simulink model "our_ch47"  (R2021a)
settings: Solver=FixedStepAuto  StartTime=0.0  StopTime=10  FixedStep=0.001  RelTol=1e-3  AbsTol=1e-3  EnableMultiTasking=on
undefined symbols (not defined in the file or in its folder): DiscIntNeverNeededParam, e2b, envs, PID_Param1, pos1, pos2, pos3, pos4, pos_load, tandem, X, x0, Y, Z
libraries: sm_lib x88, nesl_utility x25
(part 4 of 6)

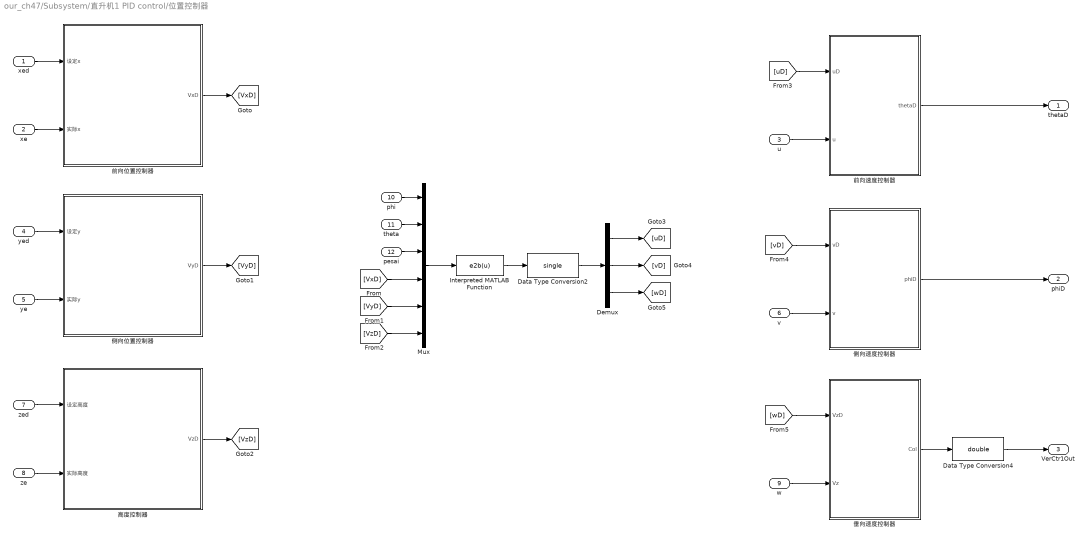
== system our_ch47/Subsystem/直升机1 PID control/位置控制器 ==
  xed : Inport
  xe : Inport  Port=2
  u : Inport  Port=3
  yed : Inport  Port=4
  ye : Inport  Port=5
  v : Inport  Port=6
  zed : Inport  Port=7
  ze : Inport  Port=8
  w : Inport  Port=9
  phi : Inport  Port=10
  theta : Inport  Port=11
  pesai : Inport  Port=12
  Data Type Conversion2 : DataTypeConversion  OutDataTypeStr=single  LockScale=on
  Data Type Conversion4 : DataTypeConversion  OutDataTypeStr=double  LockScale=on
  Demux : Demux  Outputs=3
  Interpreted MATLAB Function : MATLABFcn  MATLABFcn=e2b(u)  OutputDimensions=3
  Mux : Mux  Inputs=6
  侧向位置控制器 : Subsystem
  侧向速度控制器 : Subsystem
  前向位置控制器 : Subsystem
  前向速度控制器 : Subsystem
  垂向速度控制器 : Subsystem
  高度控制器 : Subsystem
  thetaD : Outport
  phiD : Outport  Port=2
  VerCtr1Out : Outport  Port=3
  wires:
  xe/1 -> 前向位置控制器/2(实际x)
  xed/1 -> 前向位置控制器/1(设定x)
  u/1 -> 前向速度控制器/2(u)
  前向速度控制器/1(thetaD) -> thetaD/1
  ye/1 -> 侧向位置控制器/2(实际y)
  yed/1 -> 侧向位置控制器/1(设定y)
  侧向速度控制器/1(phiD) -> phiD/1
  v/1 -> 侧向速度控制器/2(v)
  [wD] -> 垂向速度控制器/1(VzD)
  垂向速度控制器/1(Col) -> Data Type Conversion4/1
  w/1 -> 垂向速度控制器/2(Vz)
  Data Type Conversion4/1 -> VerCtr1Out/1
  zed/1 -> 高度控制器/1(设定高度)
  ze/1 -> 高度控制器/2(实际高度)
  前向位置控制器/1(VxD) -> [VxD]
  侧向位置控制器/1(VyD) -> [VyD]
  高度控制器/1(VzD) -> [VzD]
  theta/1 -> Mux/2
  phi/1 -> Mux/1
  pesai/1 -> Mux/3
  [VxD] -> Mux/4
  [VyD] -> Mux/5
  [VzD] -> Mux/6
  Interpreted MATLAB Function/1 -> Data Type Conversion2/1
  Demux/3 -> [wD]
  Demux/2 -> [vD]
  Demux/1 -> [uD]
  Data Type Conversion2/1 -> Demux/1
  Mux/1 -> Interpreted MATLAB Function/1
  [vD] -> 侧向速度控制器/1(vD)
  [uD] -> 前向速度控制器/1(uD)

== system our_ch47/Subsystem/直升机1 PID control/姿态控制器 ==
  RollD : Inport
  Roll : Inport  Port=2
  RollRate : Inport  Port=3
  PitchD : Inport  Port=4
  Pitch : Inport  Port=5
  PitchRate : Inport  Port=6
  YawD : Inport  Port=7
  Yaw : Inport  Port=8
  YawRate : Inport  Port=9
  Data Type Conversion1 : DataTypeConversion  OutDataTypeStr=double  LockScale=on
  Data Type Conversion2 : DataTypeConversion  OutDataTypeStr=double  LockScale=on
  Data Type Conversion3 : DataTypeConversion  OutDataTypeStr=double  LockScale=on
  俯仰控制器H-A : Subsystem
  滚转控制器H-A : Subsystem
  航向控制器H-A : Subsystem
  RollCtrlOut : Outport  VectorParamsAs1DForOutWhenUnconnected=off
  PitchCtrlOut : Outport  Port=2  VectorParamsAs1DForOutWhenUnconnected=off
  YawCtrlOut : Outport  Port=3  VectorParamsAs1DForOutWhenUnconnected=off
  wires:
  PitchRate/1 -> 俯仰控制器H-A/3(PitchRate)
  PitchD/1 -> 俯仰控制器H-A/1(PitchD)
  Pitch/1 -> 俯仰控制器H-A/2(Pitch)
  RollD/1 -> 滚转控制器H-A/1(RollD)
  Roll/1 -> 滚转控制器H-A/2(Roll)
  RollRate/1 -> 滚转控制器H-A/3(RollRate)
  YawRate/1 -> 航向控制器H-A/3(YawRate)
  YawD/1 -> 航向控制器H-A/1(YawD)
  Yaw/1 -> 航向控制器H-A/2(Yaw)
  俯仰控制器H-A/1(Lon) -> Data Type Conversion1/1
  航向控制器H-A/1(Ped) -> Data Type Conversion3/1
  滚转控制器H-A/1(Lat) -> Data Type Conversion2/1
  Data Type Conversion2/1 -> RollCtrlOut/1
  Data Type Conversion1/1 -> PitchCtrlOut/1
  Data Type Conversion3/1 -> YawCtrlOut/1

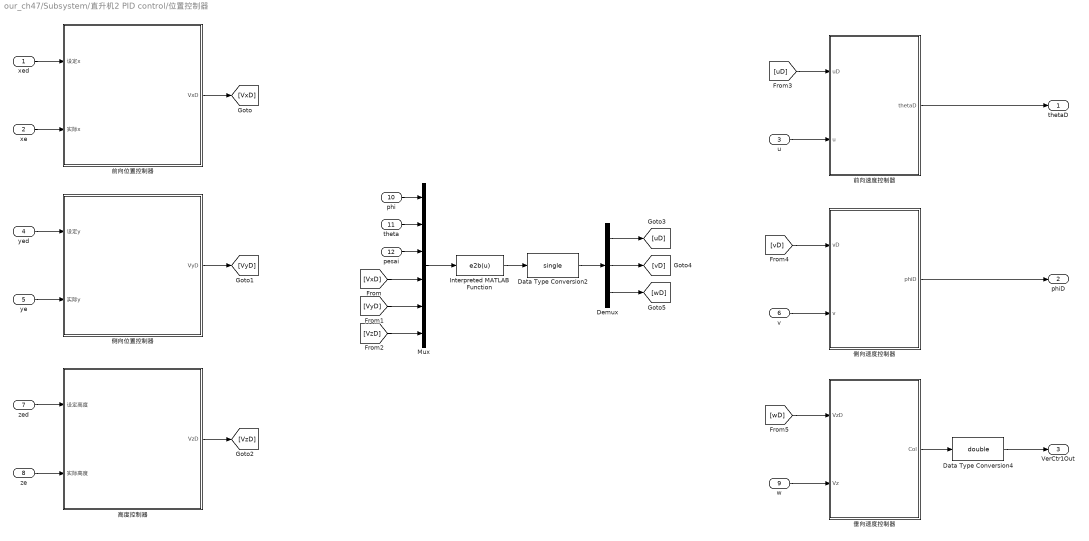
== system our_ch47/Subsystem/直升机2 PID control/位置控制器 ==
  xed : Inport
  xe : Inport  Port=2
  u : Inport  Port=3
  yed : Inport  Port=4
  ye : Inport  Port=5
  v : Inport  Port=6
  zed : Inport  Port=7
  ze : Inport  Port=8
  w : Inport  Port=9
  phi : Inport  Port=10
  theta : Inport  Port=11
  pesai : Inport  Port=12
  Data Type Conversion2 : DataTypeConversion  OutDataTypeStr=single  LockScale=on
  Data Type Conversion4 : DataTypeConversion  OutDataTypeStr=double  LockScale=on
  Demux : Demux  Outputs=3
  Interpreted MATLAB Function : MATLABFcn  MATLABFcn=e2b(u)  OutputDimensions=3
  Mux : Mux  Inputs=6
  侧向位置控制器 : Subsystem
  侧向速度控制器 : Subsystem
  前向位置控制器 : Subsystem
  前向速度控制器 : Subsystem
  垂向速度控制器 : Subsystem
  高度控制器 : Subsystem
  thetaD : Outport
  phiD : Outport  Port=2
  VerCtr1Out : Outport  Port=3
  wires:
  xe/1 -> 前向位置控制器/2(实际x)
  xed/1 -> 前向位置控制器/1(设定x)
  u/1 -> 前向速度控制器/2(u)
  前向速度控制器/1(thetaD) -> thetaD/1
  ye/1 -> 侧向位置控制器/2(实际y)
  yed/1 -> 侧向位置控制器/1(设定y)
  侧向速度控制器/1(phiD) -> phiD/1
  v/1 -> 侧向速度控制器/2(v)
  [wD] -> 垂向速度控制器/1(VzD)
  垂向速度控制器/1(Col) -> Data Type Conversion4/1
  w/1 -> 垂向速度控制器/2(Vz)
  Data Type Conversion4/1 -> VerCtr1Out/1
  zed/1 -> 高度控制器/1(设定高度)
  ze/1 -> 高度控制器/2(实际高度)
  前向位置控制器/1(VxD) -> [VxD]
  侧向位置控制器/1(VyD) -> [VyD]
  高度控制器/1(VzD) -> [VzD]
  theta/1 -> Mux/2
  phi/1 -> Mux/1
  pesai/1 -> Mux/3
  [VxD] -> Mux/4
  [VyD] -> Mux/5
  [VzD] -> Mux/6
  Interpreted MATLAB Function/1 -> Data Type Conversion2/1
  Demux/3 -> [wD]
  Demux/2 -> [vD]
  Demux/1 -> [uD]
  Data Type Conversion2/1 -> Demux/1
  Mux/1 -> Interpreted MATLAB Function/1
  [vD] -> 侧向速度控制器/1(vD)
  [uD] -> 前向速度控制器/1(uD)

== system our_ch47/Subsystem/直升机2 PID control/姿态控制器 ==
  RollD : Inport
  Roll : Inport  Port=2
  RollRate : Inport  Port=3
  PitchD : Inport  Port=4
  Pitch : Inport  Port=5
  PitchRate : Inport  Port=6
  YawD : Inport  Port=7
  Yaw : Inport  Port=8
  YawRate : Inport  Port=9
  Data Type Conversion1 : DataTypeConversion  OutDataTypeStr=double  LockScale=on
  Data Type Conversion2 : DataTypeConversion  OutDataTypeStr=double  LockScale=on
  Data Type Conversion3 : DataTypeConversion  OutDataTypeStr=double  LockScale=on
  俯仰控制器H-A : Subsystem
  滚转控制器H-A : Subsystem
  航向控制器H-A : Subsystem
  RollCtrlOut : Outport  VectorParamsAs1DForOutWhenUnconnected=off
  PitchCtrlOut : Outport  Port=2  VectorParamsAs1DForOutWhenUnconnected=off
  YawCtrlOut : Outport  Port=3  VectorParamsAs1DForOutWhenUnconnected=off
  wires:
  PitchRate/1 -> 俯仰控制器H-A/3(PitchRate)
  PitchD/1 -> 俯仰控制器H-A/1(PitchD)
  Pitch/1 -> 俯仰控制器H-A/2(Pitch)
  RollD/1 -> 滚转控制器H-A/1(RollD)
  Roll/1 -> 滚转控制器H-A/2(Roll)
  RollRate/1 -> 滚转控制器H-A/3(RollRate)
  YawRate/1 -> 航向控制器H-A/3(YawRate)
  YawD/1 -> 航向控制器H-A/1(YawD)
  Yaw/1 -> 航向控制器H-A/2(Yaw)
  俯仰控制器H-A/1(Lon) -> Data Type Conversion1/1
  航向控制器H-A/1(Ped) -> Data Type Conversion3/1
  滚转控制器H-A/1(Lat) -> Data Type Conversion2/1
  Data Type Conversion2/1 -> RollCtrlOut/1
  Data Type Conversion1/1 -> PitchCtrlOut/1
  Data Type Conversion3/1 -> YawCtrlOut/1

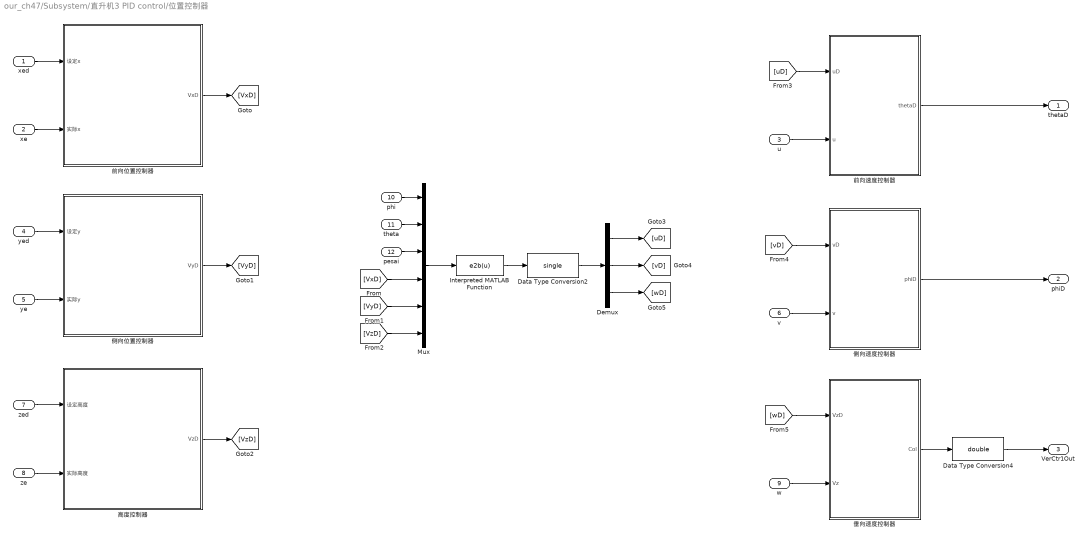
== system our_ch47/Subsystem/直升机3 PID control/位置控制器 ==
  xed : Inport
  xe : Inport  Port=2
  u : Inport  Port=3
  yed : Inport  Port=4
  ye : Inport  Port=5
  v : Inport  Port=6
  zed : Inport  Port=7
  ze : Inport  Port=8
  w : Inport  Port=9
  phi : Inport  Port=10
  theta : Inport  Port=11
  pesai : Inport  Port=12
  Data Type Conversion2 : DataTypeConversion  OutDataTypeStr=single  LockScale=on
  Data Type Conversion4 : DataTypeConversion  OutDataTypeStr=double  LockScale=on
  Demux : Demux  Outputs=3
  Interpreted MATLAB Function : MATLABFcn  MATLABFcn=e2b(u)  OutputDimensions=3
  Mux : Mux  Inputs=6
  侧向位置控制器 : Subsystem
  侧向速度控制器 : Subsystem
  前向位置控制器 : Subsystem
  前向速度控制器 : Subsystem
  垂向速度控制器 : Subsystem
  高度控制器 : Subsystem
  thetaD : Outport
  phiD : Outport  Port=2
  VerCtr1Out : Outport  Port=3
  wires:
  [uD] -> 前向速度控制器/1(uD)
  [vD] -> 侧向速度控制器/1(vD)
  Mux/1 -> Interpreted MATLAB Function/1
  Data Type Conversion2/1 -> Demux/1
  Demux/1 -> [uD]
  Demux/2 -> [vD]
  Demux/3 -> [wD]
  Interpreted MATLAB Function/1 -> Data Type Conversion2/1
  [VzD] -> Mux/6
  [VyD] -> Mux/5
  [VxD] -> Mux/4
  pesai/1 -> Mux/3
  phi/1 -> Mux/1
  theta/1 -> Mux/2
  高度控制器/1(VzD) -> [VzD]
  侧向位置控制器/1(VyD) -> [VyD]
  前向位置控制器/1(VxD) -> [VxD]
  ze/1 -> 高度控制器/2(实际高度)
  zed/1 -> 高度控制器/1(设定高度)
  Data Type Conversion4/1 -> VerCtr1Out/1
  w/1 -> 垂向速度控制器/2(Vz)
  垂向速度控制器/1(Col) -> Data Type Conversion4/1
  [wD] -> 垂向速度控制器/1(VzD)
  v/1 -> 侧向速度控制器/2(v)
  侧向速度控制器/1(phiD) -> phiD/1
  yed/1 -> 侧向位置控制器/1(设定y)
  ye/1 -> 侧向位置控制器/2(实际y)
  前向速度控制器/1(thetaD) -> thetaD/1
  u/1 -> 前向速度控制器/2(u)
  xed/1 -> 前向位置控制器/1(设定x)
  xe/1 -> 前向位置控制器/2(实际x)

== system our_ch47/Subsystem/直升机3 PID control/姿态控制器 ==
  RollD : Inport
  Roll : Inport  Port=2
  RollRate : Inport  Port=3
  PitchD : Inport  Port=4
  Pitch : Inport  Port=5
  PitchRate : Inport  Port=6
  YawD : Inport  Port=7
  Yaw : Inport  Port=8
  YawRate : Inport  Port=9
  Data Type Conversion1 : DataTypeConversion  OutDataTypeStr=double  LockScale=on
  Data Type Conversion2 : DataTypeConversion  OutDataTypeStr=double  LockScale=on
  Data Type Conversion3 : DataTypeConversion  OutDataTypeStr=double  LockScale=on
  俯仰控制器H-A : Subsystem
  滚转控制器H-A : Subsystem
  航向控制器H-A : Subsystem
  RollCtrlOut : Outport  VectorParamsAs1DForOutWhenUnconnected=off
  PitchCtrlOut : Outport  Port=2  VectorParamsAs1DForOutWhenUnconnected=off
  YawCtrlOut : Outport  Port=3  VectorParamsAs1DForOutWhenUnconnected=off
  wires:
  Data Type Conversion3/1 -> YawCtrlOut/1
  Data Type Conversion1/1 -> PitchCtrlOut/1
  Data Type Conversion2/1 -> RollCtrlOut/1
  滚转控制器H-A/1(Lat) -> Data Type Conversion2/1
  航向控制器H-A/1(Ped) -> Data Type Conversion3/1
  俯仰控制器H-A/1(Lon) -> Data Type Conversion1/1
  Yaw/1 -> 航向控制器H-A/2(Yaw)
  YawD/1 -> 航向控制器H-A/1(YawD)
  YawRate/1 -> 航向控制器H-A/3(YawRate)
  RollRate/1 -> 滚转控制器H-A/3(RollRate)
  Roll/1 -> 滚转控制器H-A/2(Roll)
  RollD/1 -> 滚转控制器H-A/1(RollD)
  Pitch/1 -> 俯仰控制器H-A/2(Pitch)
  PitchD/1 -> 俯仰控制器H-A/1(PitchD)
  PitchRate/1 -> 俯仰控制器H-A/3(PitchRate)

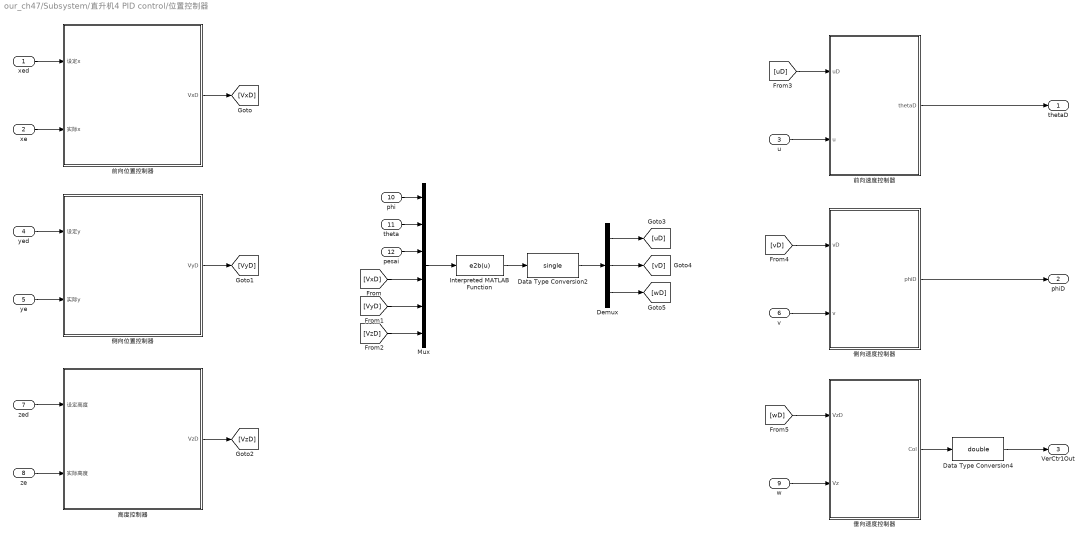
== system our_ch47/Subsystem/直升机4 PID control/位置控制器 ==
  xed : Inport
  xe : Inport  Port=2
  u : Inport  Port=3
  yed : Inport  Port=4
  ye : Inport  Port=5
  v : Inport  Port=6
  zed : Inport  Port=7
  ze : Inport  Port=8
  w : Inport  Port=9
  phi : Inport  Port=10
  theta : Inport  Port=11
  pesai : Inport  Port=12
  Data Type Conversion2 : DataTypeConversion  OutDataTypeStr=single  LockScale=on
  Data Type Conversion4 : DataTypeConversion  OutDataTypeStr=double  LockScale=on
  Demux : Demux  Outputs=3
  Interpreted MATLAB Function : MATLABFcn  MATLABFcn=e2b(u)  OutputDimensions=3
  Mux : Mux  Inputs=6
  侧向位置控制器 : Subsystem
  侧向速度控制器 : Subsystem
  前向位置控制器 : Subsystem
  前向速度控制器 : Subsystem
  垂向速度控制器 : Subsystem
  高度控制器 : Subsystem
  thetaD : Outport
  phiD : Outport  Port=2
  VerCtr1Out : Outport  Port=3
  wires:
  xe/1 -> 前向位置控制器/2(实际x)
  xed/1 -> 前向位置控制器/1(设定x)
  u/1 -> 前向速度控制器/2(u)
  前向速度控制器/1(thetaD) -> thetaD/1
  ye/1 -> 侧向位置控制器/2(实际y)
  yed/1 -> 侧向位置控制器/1(设定y)
  侧向速度控制器/1(phiD) -> phiD/1
  v/1 -> 侧向速度控制器/2(v)
  [wD] -> 垂向速度控制器/1(VzD)
  垂向速度控制器/1(Col) -> Data Type Conversion4/1
  w/1 -> 垂向速度控制器/2(Vz)
  Data Type Conversion4/1 -> VerCtr1Out/1
  zed/1 -> 高度控制器/1(设定高度)
  ze/1 -> 高度控制器/2(实际高度)
  前向位置控制器/1(VxD) -> [VxD]
  侧向位置控制器/1(VyD) -> [VyD]
  高度控制器/1(VzD) -> [VzD]
  theta/1 -> Mux/2
  phi/1 -> Mux/1
  pesai/1 -> Mux/3
  [VxD] -> Mux/4
  [VyD] -> Mux/5
  [VzD] -> Mux/6
  Interpreted MATLAB Function/1 -> Data Type Conversion2/1
  Demux/3 -> [wD]
  Demux/2 -> [vD]
  Demux/1 -> [uD]
  Data Type Conversion2/1 -> Demux/1
  Mux/1 -> Interpreted MATLAB Function/1
  [vD] -> 侧向速度控制器/1(vD)
  [uD] -> 前向速度控制器/1(uD)

== system our_ch47/Subsystem/直升机4 PID control/姿态控制器 ==
  RollD : Inport
  Roll : Inport  Port=2
  RollRate : Inport  Port=3
  PitchD : Inport  Port=4
  Pitch : Inport  Port=5
  PitchRate : Inport  Port=6
  YawD : Inport  Port=7
  Yaw : Inport  Port=8
  YawRate : Inport  Port=9
  Data Type Conversion1 : DataTypeConversion  OutDataTypeStr=double  LockScale=on
  Data Type Conversion2 : DataTypeConversion  OutDataTypeStr=double  LockScale=on
  Data Type Conversion3 : DataTypeConversion  OutDataTypeStr=double  LockScale=on
  俯仰控制器H-A : Subsystem
  滚转控制器H-A : Subsystem
  航向控制器H-A : Subsystem
  RollCtrlOut : Outport  VectorParamsAs1DForOutWhenUnconnected=off
  PitchCtrlOut : Outport  Port=2  VectorParamsAs1DForOutWhenUnconnected=off
  YawCtrlOut : Outport  Port=3  VectorParamsAs1DForOutWhenUnconnected=off
  wires:
  PitchRate/1 -> 俯仰控制器H-A/3(PitchRate)
  PitchD/1 -> 俯仰控制器H-A/1(PitchD)
  Pitch/1 -> 俯仰控制器H-A/2(Pitch)
  RollD/1 -> 滚转控制器H-A/1(RollD)
  Roll/1 -> 滚转控制器H-A/2(Roll)
  RollRate/1 -> 滚转控制器H-A/3(RollRate)
  YawRate/1 -> 航向控制器H-A/3(YawRate)
  YawD/1 -> 航向控制器H-A/1(YawD)
  Yaw/1 -> 航向控制器H-A/2(Yaw)
  俯仰控制器H-A/1(Lon) -> Data Type Conversion1/1
  航向控制器H-A/1(Ped) -> Data Type Conversion3/1
  滚转控制器H-A/1(Lat) -> Data Type Conversion2/1
  Data Type Conversion2/1 -> RollCtrlOut/1
  Data Type Conversion1/1 -> PitchCtrlOut/1
  Data Type Conversion3/1 -> YawCtrlOut/1

== system our_ch47/Subsystem/直升机1 PID control/位置控制器/侧向位置控制器 ==
  设定y : Inport
  实际y : Inport  Port=2
  Data Type Conversion1 : DataTypeConversion  OutDataTypeStr=single  LockScale=on
  Data Type Conversion2 : DataTypeConversion  OutDataTypeStr=single  LockScale=on
  Data Type Conversion3 : DataTypeConversion  OutDataTypeStr=double  LockScale=on
  侧向位置控制器 : Subsystem
  VyD : Outport
  wires:
  设定y/1 -> Data Type Conversion1/1
  实际y/1 -> Data Type Conversion2/1
  侧向位置控制器/1(VyD) -> Data Type Conversion3/1
  Data Type Conversion1/1 -> 侧向位置控制器/1(yd_m)
  Data Type Conversion2/1 -> 侧向位置控制器/2(y_m)
  Data Type Conversion3/1 -> VyD/1

== system our_ch47/Subsystem/直升机1 PID control/位置控制器/侧向速度控制器 ==
  vD : Inport
  v : Inport  Port=2
  Constant : Constant  Value=0  OutDataTypeStr=Inherit: Inherit via back propagation
  Data Type Conversion : DataTypeConversion  OutDataTypeStr=double
  PID_Controller : Subsystem
  Saturation : Saturate  UpperLimit=15  LowerLimit=-15
  Subtract : Sum  Inputs=+-
  phiD : Outport  VectorParamsAs1DForOutWhenUnconnected=off
  wires:
  Saturation/1 -> Data Type Conversion/1
  PID_Controller/1(u) -> Saturation/1
  Data Type Conversion/1 -> phiD/1
  Constant/1 -> PID_Controller/2(reset)
  Subtract/1 -> PID_Controller/1(err)
  v/1 -> Subtract/2
  vD/1 -> Subtract/1

== system our_ch47/Subsystem/直升机1 PID control/位置控制器/前向位置控制器 ==
  设定x : Inport
  实际x : Inport  Port=2
  Data Type Conversion1 : DataTypeConversion  OutDataTypeStr=single  LockScale=on
  Data Type Conversion2 : DataTypeConversion  OutDataTypeStr=single  LockScale=on
  Data Type Conversion3 : DataTypeConversion  OutDataTypeStr=double  LockScale=on
  前向位置控制器 : Subsystem
  VxD : Outport
  wires:
  实际x/1 -> Data Type Conversion1/1
  设定x/1 -> Data Type Conversion2/1
  Data Type Conversion1/1 -> 前向位置控制器/2(x_m)
  Data Type Conversion2/1 -> 前向位置控制器/1(xd_m)
  前向位置控制器/1(VxD) -> Data Type Conversion3/1
  Data Type Conversion3/1 -> VxD/1

== system our_ch47/Subsystem/直升机1 PID control/位置控制器/前向速度控制器 ==
  uD : Inport
  u : Inport  Port=2
  Constant : Constant  Value=0  OutDataTypeStr=Inherit: Inherit via back propagation
  Gain : Gain  Gain=-1
  PID_Controller : Subsystem
  Saturation : Saturate  UpperLimit=15  LowerLimit=-15
  Subtract : Sum  Inputs=+-
  thetaD : Outport  VectorParamsAs1DForOutWhenUnconnected=off
  wires:
  uD/1 -> Subtract/1
  u/1 -> Subtract/2
  Subtract/1 -> PID_Controller/1(err)
  Constant/1 -> PID_Controller/2(reset)
  PID_Controller/1(u) -> Saturation/1
  Saturation/1 -> Gain/1
  Gain/1 -> thetaD/1

== system our_ch47/Subsystem/直升机1 PID control/位置控制器/垂向速度控制器 ==
  VzD : Inport
  Vz : Inport  Port=2
  Constant : Constant  Value=0  OutDataTypeStr=Inherit: Inherit via back propagation
  Data Type Conversion : DataTypeConversion  OutDataTypeStr=double
  Gain : Gain  Gain=-1
  PID_Controller : Subsystem
  Saturation : Saturate  UpperLimit=8  LowerLimit=-6
  Subtract : Sum  Inputs=+-
  Sum : Sum  Inputs=|++
  hover_throttle : Constant  Value=x0(1)  OutDataTypeStr=Inherit: Inherit via back propagation
  Col : Outport  VectorParamsAs1DForOutWhenUnconnected=off
  wires:
  VzD/1 -> Subtract/1
  Vz/1 -> Subtract/2
  Subtract/1 -> PID_Controller/1(err)
  Constant/1 -> PID_Controller/2(reset)
  Data Type Conversion/1 -> Col/1
  hover_throttle/1 -> Sum/2
  PID_Controller/1(u) -> Saturation/1
  Saturation/1 -> Gain/1
  Sum/1 -> Data Type Conversion/1
  Gain/1 -> Sum/1

== system our_ch47/Subsystem/直升机1 PID control/位置控制器/高度控制器 ==
  设定高度 : Inport
  实际高度 : Inport  Port=2
  Data Type Conversion1 : DataTypeConversion  OutDataTypeStr=single  LockScale=on
  Data Type Conversion2 : DataTypeConversion  OutDataTypeStr=single  LockScale=on
  Data Type Conversion3 : DataTypeConversion  OutDataTypeStr=double  LockScale=on
  高度控制器H-A : Subsystem
  VzD : Outport
  wires:
  实际高度/1 -> Data Type Conversion2/1
  设定高度/1 -> Data Type Conversion1/1
  高度控制器H-A/1(VzD) -> Data Type Conversion3/1
  Data Type Conversion1/1 -> 高度控制器H-A/1(altitude_sp_m)
  Data Type Conversion2/1 -> 高度控制器H-A/2(altitude_m)
  Data Type Conversion3/1 -> VzD/1

== system our_ch47/Subsystem/直升机1 PID control/姿态控制器/俯仰控制器H-A ==
  PitchD : Inport
  Pitch : Inport  Port=2
  PitchRate : Inport  Port=3
  AltitudeV_Controller : Subsystem
  Data Type Conversion : DataTypeConversion  OutDataTypeStr=single  LockScale=on
  Data Type Conversion1 : DataTypeConversion  OutDataTypeStr=single  LockScale=on
  角度换 : Subsystem
  Lon : Outport  VectorParamsAs1DForOutWhenUnconnected=off
  wires:
  AltitudeV_Controller/1(Lon) -> Lon/1
  PitchRate/1 -> Data Type Conversion1/1
  Pitch/1 -> Data Type Conversion/1
  PitchD/1 -> 角度换/1(PitchD)
  Data Type Conversion/1 -> 角度换/2(Pitch)
  Data Type Conversion1/1 -> AltitudeV_Controller/2(PitchRate)
  角度换/1(PitchRateD) -> AltitudeV_Controller/1(PitchRateD)

== system our_ch47/Subsystem/直升机1 PID control/姿态控制器/滚转控制器H-A ==
  RollD : Inport
  Roll : Inport  Port=2
  RollRate : Inport  Port=3
  AltitudeV_Controller : Subsystem
  Altitude_Controller : Subsystem
  Data Type Conversion : DataTypeConversion  OutDataTypeStr=single  LockScale=on
  Data Type Conversion1 : DataTypeConversion  OutDataTypeStr=single  LockScale=on
  Lat : Outport  VectorParamsAs1DForOutWhenUnconnected=off
  wires:
  AltitudeV_Controller/1(Lat) -> Lat/1  "lat"
  RollRate/1 -> Data Type Conversion1/1
  Roll/1 -> Data Type Conversion/1
  Data Type Conversion/1 -> Altitude_Controller/2(Roll)
  Data Type Conversion1/1 -> AltitudeV_Controller/2(RollRate)
  RollD/1 -> Altitude_Controller/1(RollD)
  Altitude_Controller/1(RollRateD) -> AltitudeV_Controller/1(RollRateD)

== system our_ch47/Subsystem/直升机1 PID control/姿态控制器/航向控制器H-A ==
  YawD : Inport
  Yaw : Inport  Port=2
  YawRate : Inport  Port=3
  AltitudeV_Controller : Subsystem
  Altitude_Controller : Subsystem
  Data Type Conversion : DataTypeConversion  OutDataTypeStr=single  LockScale=on
  Data Type Conversion1 : DataTypeConversion  OutDataTypeStr=single  LockScale=on
  Ped : Outport  VectorParamsAs1DForOutWhenUnconnected=off
  wires:
  AltitudeV_Controller/1(Ped) -> Ped/1
  YawRate/1 -> Data Type Conversion1/1
  Yaw/1 -> Data Type Conversion/1
  YawD/1 -> Altitude_Controller/1(YawD)
  Data Type Conversion/1 -> Altitude_Controller/2(Yaw)
  Data Type Conversion1/1 -> AltitudeV_Controller/2(YawRate)
  Altitude_Controller/1(YawRateD) -> AltitudeV_Controller/1(YawRateD)

== system our_ch47/Subsystem/直升机2 PID control/位置控制器/侧向位置控制器 ==
  设定y : Inport
  实际y : Inport  Port=2
  Data Type Conversion1 : DataTypeConversion  OutDataTypeStr=single  LockScale=on
  Data Type Conversion2 : DataTypeConversion  OutDataTypeStr=single  LockScale=on
  Data Type Conversion3 : DataTypeConversion  OutDataTypeStr=double  LockScale=on
  侧向位置控制器 : Subsystem
  VyD : Outport
  wires:
  设定y/1 -> Data Type Conversion1/1
  实际y/1 -> Data Type Conversion2/1
  侧向位置控制器/1(VyD) -> Data Type Conversion3/1
  Data Type Conversion1/1 -> 侧向位置控制器/1(yd_m)
  Data Type Conversion2/1 -> 侧向位置控制器/2(y_m)
  Data Type Conversion3/1 -> VyD/1

== system our_ch47/Subsystem/直升机2 PID control/位置控制器/侧向速度控制器 ==
  vD : Inport
  v : Inport  Port=2
  Constant : Constant  Value=0  OutDataTypeStr=Inherit: Inherit via back propagation
  Data Type Conversion : DataTypeConversion  OutDataTypeStr=double
  PID_Controller : Subsystem
  Saturation : Saturate  UpperLimit=15  LowerLimit=-15
  Subtract : Sum  Inputs=+-
  phiD : Outport  VectorParamsAs1DForOutWhenUnconnected=off
  wires:
  Saturation/1 -> Data Type Conversion/1
  PID_Controller/1(u) -> Saturation/1
  Data Type Conversion/1 -> phiD/1
  Constant/1 -> PID_Controller/2(reset)
  Subtract/1 -> PID_Controller/1(err)
  v/1 -> Subtract/2
  vD/1 -> Subtract/1

== system our_ch47/Subsystem/直升机2 PID control/位置控制器/前向位置控制器 ==
  设定x : Inport
  实际x : Inport  Port=2
  Data Type Conversion1 : DataTypeConversion  OutDataTypeStr=single  LockScale=on
  Data Type Conversion2 : DataTypeConversion  OutDataTypeStr=single  LockScale=on
  Data Type Conversion3 : DataTypeConversion  OutDataTypeStr=double  LockScale=on
  前向位置控制器 : Subsystem
  VxD : Outport
  wires:
  实际x/1 -> Data Type Conversion1/1
  设定x/1 -> Data Type Conversion2/1
  Data Type Conversion1/1 -> 前向位置控制器/2(x_m)
  Data Type Conversion2/1 -> 前向位置控制器/1(xd_m)
  前向位置控制器/1(VxD) -> Data Type Conversion3/1
  Data Type Conversion3/1 -> VxD/1

== system our_ch47/Subsystem/直升机2 PID control/位置控制器/前向速度控制器 ==
  uD : Inport
  u : Inport  Port=2
  Constant : Constant  Value=0  OutDataTypeStr=Inherit: Inherit via back propagation
  Gain : Gain  Gain=-1
  PID_Controller : Subsystem
  Saturation : Saturate  UpperLimit=15  LowerLimit=-15
  Subtract : Sum  Inputs=+-
  thetaD : Outport  VectorParamsAs1DForOutWhenUnconnected=off
  wires:
  uD/1 -> Subtract/1
  u/1 -> Subtract/2
  Subtract/1 -> PID_Controller/1(err)
  Constant/1 -> PID_Controller/2(reset)
  PID_Controller/1(u) -> Saturation/1
  Saturation/1 -> Gain/1
  Gain/1 -> thetaD/1

== system our_ch47/Subsystem/直升机2 PID control/位置控制器/垂向速度控制器 ==
  VzD : Inport
  Vz : Inport  Port=2
  Constant : Constant  Value=0  OutDataTypeStr=Inherit: Inherit via back propagation
  Data Type Conversion : DataTypeConversion  OutDataTypeStr=double
  Gain : Gain  Gain=-1
  PID_Controller : Subsystem
  Saturation : Saturate  UpperLimit=8  LowerLimit=-6
  Subtract : Sum  Inputs=+-
  Sum : Sum  Inputs=|++
  hover_throttle : Constant  Value=x0(1)  OutDataTypeStr=Inherit: Inherit via back propagation
  Col : Outport  VectorParamsAs1DForOutWhenUnconnected=off
  wires:
  VzD/1 -> Subtract/1
  Vz/1 -> Subtract/2
  Subtract/1 -> PID_Controller/1(err)
  Constant/1 -> PID_Controller/2(reset)
  Data Type Conversion/1 -> Col/1
  hover_throttle/1 -> Sum/2
  PID_Controller/1(u) -> Saturation/1
  Saturation/1 -> Gain/1
  Sum/1 -> Data Type Conversion/1
  Gain/1 -> Sum/1

== system our_ch47/Subsystem/直升机2 PID control/位置控制器/高度控制器 ==
  设定高度 : Inport
  实际高度 : Inport  Port=2
  Data Type Conversion1 : DataTypeConversion  OutDataTypeStr=single  LockScale=on
  Data Type Conversion2 : DataTypeConversion  OutDataTypeStr=single  LockScale=on
  Data Type Conversion3 : DataTypeConversion  OutDataTypeStr=double  LockScale=on
  高度控制器H-A : Subsystem
  VzD : Outport
  wires:
  实际高度/1 -> Data Type Conversion2/1
  设定高度/1 -> Data Type Conversion1/1
  高度控制器H-A/1(VzD) -> Data Type Conversion3/1
  Data Type Conversion1/1 -> 高度控制器H-A/1(altitude_sp_m)
  Data Type Conversion2/1 -> 高度控制器H-A/2(altitude_m)
  Data Type Conversion3/1 -> VzD/1

== system our_ch47/Subsystem/直升机2 PID control/姿态控制器/俯仰控制器H-A ==
  PitchD : Inport
  Pitch : Inport  Port=2
  PitchRate : Inport  Port=3
  AltitudeV_Controller : Subsystem
  Data Type Conversion : DataTypeConversion  OutDataTypeStr=single  LockScale=on
  Data Type Conversion1 : DataTypeConversion  OutDataTypeStr=single  LockScale=on
  角度换 : Subsystem
  Lon : Outport  VectorParamsAs1DForOutWhenUnconnected=off
  wires:
  AltitudeV_Controller/1(Lon) -> Lon/1
  PitchRate/1 -> Data Type Conversion1/1
  Pitch/1 -> Data Type Conversion/1
  PitchD/1 -> 角度换/1(PitchD)
  Data Type Conversion/1 -> 角度换/2(Pitch)
  Data Type Conversion1/1 -> AltitudeV_Controller/2(PitchRate)
  角度换/1(PitchRateD) -> AltitudeV_Controller/1(PitchRateD)

== system our_ch47/Subsystem/直升机2 PID control/姿态控制器/滚转控制器H-A ==
  RollD : Inport
  Roll : Inport  Port=2
  RollRate : Inport  Port=3
  AltitudeV_Controller : Subsystem
  Altitude_Controller : Subsystem
  Data Type Conversion : DataTypeConversion  OutDataTypeStr=single  LockScale=on
  Data Type Conversion1 : DataTypeConversion  OutDataTypeStr=single  LockScale=on
  Lat : Outport  VectorParamsAs1DForOutWhenUnconnected=off
  wires:
  AltitudeV_Controller/1(Lat) -> Lat/1  "lat"
  RollRate/1 -> Data Type Conversion1/1
  Roll/1 -> Data Type Conversion/1
  Data Type Conversion/1 -> Altitude_Controller/2(Roll)
  Data Type Conversion1/1 -> AltitudeV_Controller/2(RollRate)
  RollD/1 -> Altitude_Controller/1(RollD)
  Altitude_Controller/1(RollRateD) -> AltitudeV_Controller/1(RollRateD)

== system our_ch47/Subsystem/直升机2 PID control/姿态控制器/航向控制器H-A ==
  YawD : Inport
  Yaw : Inport  Port=2
  YawRate : Inport  Port=3
  AltitudeV_Controller : Subsystem
  Altitude_Controller : Subsystem
  Data Type Conversion : DataTypeConversion  OutDataTypeStr=single  LockScale=on
  Data Type Conversion1 : DataTypeConversion  OutDataTypeStr=single  LockScale=on
  Ped : Outport  VectorParamsAs1DForOutWhenUnconnected=off
  wires:
  AltitudeV_Controller/1(Ped) -> Ped/1
  YawRate/1 -> Data Type Conversion1/1
  Yaw/1 -> Data Type Conversion/1
  YawD/1 -> Altitude_Controller/1(YawD)
  Data Type Conversion/1 -> Altitude_Controller/2(Yaw)
  Data Type Conversion1/1 -> AltitudeV_Controller/2(YawRate)
  Altitude_Controller/1(YawRateD) -> AltitudeV_Controller/1(YawRateD)

== system our_ch47/Subsystem/直升机3 PID control/位置控制器/侧向位置控制器 ==
  设定y : Inport
  实际y : Inport  Port=2
  Data Type Conversion1 : DataTypeConversion  OutDataTypeStr=single  LockScale=on
  Data Type Conversion2 : DataTypeConversion  OutDataTypeStr=single  LockScale=on
  Data Type Conversion3 : DataTypeConversion  OutDataTypeStr=double  LockScale=on
  侧向位置控制器 : Subsystem
  VyD : Outport
  wires:
  Data Type Conversion3/1 -> VyD/1
  Data Type Conversion2/1 -> 侧向位置控制器/2(y_m)
  Data Type Conversion1/1 -> 侧向位置控制器/1(yd_m)
  侧向位置控制器/1(VyD) -> Data Type Conversion3/1
  实际y/1 -> Data Type Conversion2/1
  设定y/1 -> Data Type Conversion1/1

== system our_ch47/Subsystem/直升机3 PID control/位置控制器/侧向速度控制器 ==
  vD : Inport
  v : Inport  Port=2
  Constant : Constant  Value=0  OutDataTypeStr=Inherit: Inherit via back propagation
  Data Type Conversion : DataTypeConversion  OutDataTypeStr=double
  PID_Controller : Subsystem
  Saturation : Saturate  UpperLimit=15  LowerLimit=-15
  Subtract : Sum  Inputs=+-
  phiD : Outport  VectorParamsAs1DForOutWhenUnconnected=off
  wires:
  vD/1 -> Subtract/1
  v/1 -> Subtract/2
  Subtract/1 -> PID_Controller/1(err)
  Constant/1 -> PID_Controller/2(reset)
  Data Type Conversion/1 -> phiD/1
  PID_Controller/1(u) -> Saturation/1
  Saturation/1 -> Data Type Conversion/1

== system our_ch47/Subsystem/直升机3 PID control/位置控制器/前向位置控制器 ==
  设定x : Inport
  实际x : Inport  Port=2
  Data Type Conversion1 : DataTypeConversion  OutDataTypeStr=single  LockScale=on
  Data Type Conversion2 : DataTypeConversion  OutDataTypeStr=single  LockScale=on
  Data Type Conversion3 : DataTypeConversion  OutDataTypeStr=double  LockScale=on
  前向位置控制器 : Subsystem
  VxD : Outport
  wires:
  Data Type Conversion3/1 -> VxD/1
  前向位置控制器/1(VxD) -> Data Type Conversion3/1
  Data Type Conversion2/1 -> 前向位置控制器/1(xd_m)
  Data Type Conversion1/1 -> 前向位置控制器/2(x_m)
  设定x/1 -> Data Type Conversion2/1
  实际x/1 -> Data Type Conversion1/1

== system our_ch47/Subsystem/直升机3 PID control/位置控制器/前向速度控制器 ==
  uD : Inport
  u : Inport  Port=2
  Constant : Constant  Value=0  OutDataTypeStr=Inherit: Inherit via back propagation
  Gain : Gain  Gain=-1
  PID_Controller : Subsystem
  Saturation : Saturate  UpperLimit=15  LowerLimit=-15
  Subtract : Sum  Inputs=+-
  thetaD : Outport  VectorParamsAs1DForOutWhenUnconnected=off
  wires:
  Gain/1 -> thetaD/1
  Saturation/1 -> Gain/1
  PID_Controller/1(u) -> Saturation/1
  Constant/1 -> PID_Controller/2(reset)
  Subtract/1 -> PID_Controller/1(err)
  u/1 -> Subtract/2
  uD/1 -> Subtract/1

== system our_ch47/Subsystem/直升机3 PID control/位置控制器/垂向速度控制器 ==
  VzD : Inport
  Vz : Inport  Port=2
  Constant : Constant  Value=0  OutDataTypeStr=Inherit: Inherit via back propagation
  Data Type Conversion : DataTypeConversion  OutDataTypeStr=double
  Gain : Gain  Gain=-1
  PID_Controller : Subsystem
  Saturation : Saturate  UpperLimit=8  LowerLimit=-6
  Subtract : Sum  Inputs=+-
  Sum : Sum  Inputs=|++
  hover_throttle : Constant  Value=x0(1)  OutDataTypeStr=Inherit: Inherit via back propagation
  Col : Outport  VectorParamsAs1DForOutWhenUnconnected=off
  wires:
  Gain/1 -> Sum/1
  Sum/1 -> Data Type Conversion/1
  Saturation/1 -> Gain/1
  PID_Controller/1(u) -> Saturation/1
  hover_throttle/1 -> Sum/2
  Data Type Conversion/1 -> Col/1
  Constant/1 -> PID_Controller/2(reset)
  Subtract/1 -> PID_Controller/1(err)
  Vz/1 -> Subtract/2
  VzD/1 -> Subtract/1

== system our_ch47/Subsystem/直升机3 PID control/位置控制器/高度控制器 ==
  设定高度 : Inport
  实际高度 : Inport  Port=2
  Data Type Conversion1 : DataTypeConversion  OutDataTypeStr=single  LockScale=on
  Data Type Conversion2 : DataTypeConversion  OutDataTypeStr=single  LockScale=on
  Data Type Conversion3 : DataTypeConversion  OutDataTypeStr=double  LockScale=on
  高度控制器H-A : Subsystem
  VzD : Outport
  wires:
  Data Type Conversion3/1 -> VzD/1
  Data Type Conversion2/1 -> 高度控制器H-A/2(altitude_m)
  Data Type Conversion1/1 -> 高度控制器H-A/1(altitude_sp_m)
  高度控制器H-A/1(VzD) -> Data Type Conversion3/1
  设定高度/1 -> Data Type Conversion1/1
  实际高度/1 -> Data Type Conversion2/1

== system our_ch47/Subsystem/直升机3 PID control/姿态控制器/俯仰控制器H-A ==
  PitchD : Inport
  Pitch : Inport  Port=2
  PitchRate : Inport  Port=3
  AltitudeV_Controller : Subsystem
  Data Type Conversion : DataTypeConversion  OutDataTypeStr=single  LockScale=on
  Data Type Conversion1 : DataTypeConversion  OutDataTypeStr=single  LockScale=on
  角度换 : Subsystem
  Lon : Outport  VectorParamsAs1DForOutWhenUnconnected=off
  wires:
  角度换/1(PitchRateD) -> AltitudeV_Controller/1(PitchRateD)
  Data Type Conversion1/1 -> AltitudeV_Controller/2(PitchRate)
  Data Type Conversion/1 -> 角度换/2(Pitch)
  PitchD/1 -> 角度换/1(PitchD)
  Pitch/1 -> Data Type Conversion/1
  PitchRate/1 -> Data Type Conversion1/1
  AltitudeV_Controller/1(Lon) -> Lon/1

== system our_ch47/Subsystem/直升机3 PID control/姿态控制器/滚转控制器H-A ==
  RollD : Inport
  Roll : Inport  Port=2
  RollRate : Inport  Port=3
  AltitudeV_Controller : Subsystem
  Altitude_Controller : Subsystem
  Data Type Conversion : DataTypeConversion  OutDataTypeStr=single  LockScale=on
  Data Type Conversion1 : DataTypeConversion  OutDataTypeStr=single  LockScale=on
  Lat : Outport  VectorParamsAs1DForOutWhenUnconnected=off
  wires:
  Altitude_Controller/1(RollRateD) -> AltitudeV_Controller/1(RollRateD)
  RollD/1 -> Altitude_Controller/1(RollD)
  Data Type Conversion1/1 -> AltitudeV_Controller/2(RollRate)
  Data Type Conversion/1 -> Altitude_Controller/2(Roll)
  Roll/1 -> Data Type Conversion/1
  RollRate/1 -> Data Type Conversion1/1
  AltitudeV_Controller/1(Lat) -> Lat/1  "lat"

== system our_ch47/Subsystem/直升机3 PID control/姿态控制器/航向控制器H-A ==
  YawD : Inport
  Yaw : Inport  Port=2
  YawRate : Inport  Port=3
  AltitudeV_Controller : Subsystem
  Altitude_Controller : Subsystem
  Data Type Conversion : DataTypeConversion  OutDataTypeStr=single  LockScale=on
  Data Type Conversion1 : DataTypeConversion  OutDataTypeStr=single  LockScale=on
  Ped : Outport  VectorParamsAs1DForOutWhenUnconnected=off
  wires:
  Altitude_Controller/1(YawRateD) -> AltitudeV_Controller/1(YawRateD)
  Data Type Conversion1/1 -> AltitudeV_Controller/2(YawRate)
  Data Type Conversion/1 -> Altitude_Controller/2(Yaw)
  YawD/1 -> Altitude_Controller/1(YawD)
  Yaw/1 -> Data Type Conversion/1
  YawRate/1 -> Data Type Conversion1/1
  AltitudeV_Controller/1(Ped) -> Ped/1

== system our_ch47/Subsystem/直升机4 PID control/位置控制器/侧向位置控制器 ==
  设定y : Inport
  实际y : Inport  Port=2
  Data Type Conversion1 : DataTypeConversion  OutDataTypeStr=single  LockScale=on
  Data Type Conversion2 : DataTypeConversion  OutDataTypeStr=single  LockScale=on
  Data Type Conversion3 : DataTypeConversion  OutDataTypeStr=double  LockScale=on
  侧向位置控制器 : Subsystem
  VyD : Outport
  wires:
  设定y/1 -> Data Type Conversion1/1
  实际y/1 -> Data Type Conversion2/1
  侧向位置控制器/1(VyD) -> Data Type Conversion3/1
  Data Type Conversion1/1 -> 侧向位置控制器/1(yd_m)
  Data Type Conversion2/1 -> 侧向位置控制器/2(y_m)
  Data Type Conversion3/1 -> VyD/1

== system our_ch47/Subsystem/直升机4 PID control/位置控制器/侧向速度控制器 ==
  vD : Inport
  v : Inport  Port=2
  Constant : Constant  Value=0  OutDataTypeStr=Inherit: Inherit via back propagation
  Data Type Conversion : DataTypeConversion  OutDataTypeStr=double
  PID_Controller : Subsystem
  Saturation : Saturate  UpperLimit=15  LowerLimit=-15
  Subtract : Sum  Inputs=+-
  phiD : Outport  VectorParamsAs1DForOutWhenUnconnected=off
  wires:
  Saturation/1 -> Data Type Conversion/1
  PID_Controller/1(u) -> Saturation/1
  Data Type Conversion/1 -> phiD/1
  Constant/1 -> PID_Controller/2(reset)
  Subtract/1 -> PID_Controller/1(err)
  v/1 -> Subtract/2
  vD/1 -> Subtract/1

== system our_ch47/Subsystem/直升机4 PID control/位置控制器/前向位置控制器 ==
  设定x : Inport
  实际x : Inport  Port=2
  Data Type Conversion1 : DataTypeConversion  OutDataTypeStr=single  LockScale=on
  Data Type Conversion2 : DataTypeConversion  OutDataTypeStr=single  LockScale=on
  Data Type Conversion3 : DataTypeConversion  OutDataTypeStr=double  LockScale=on
  前向位置控制器 : Subsystem
  VxD : Outport
  wires:
  实际x/1 -> Data Type Conversion1/1
  设定x/1 -> Data Type Conversion2/1
  Data Type Conversion1/1 -> 前向位置控制器/2(x_m)
  Data Type Conversion2/1 -> 前向位置控制器/1(xd_m)
  前向位置控制器/1(VxD) -> Data Type Conversion3/1
  Data Type Conversion3/1 -> VxD/1

== system our_ch47/Subsystem/直升机4 PID control/位置控制器/前向速度控制器 ==
  uD : Inport
  u : Inport  Port=2
  Constant : Constant  Value=0  OutDataTypeStr=Inherit: Inherit via back propagation
  Gain : Gain  Gain=-1
  PID_Controller : Subsystem
  Saturation : Saturate  UpperLimit=15  LowerLimit=-15
  Subtract : Sum  Inputs=+-
  thetaD : Outport  VectorParamsAs1DForOutWhenUnconnected=off
  wires:
  uD/1 -> Subtract/1
  u/1 -> Subtract/2
  Subtract/1 -> PID_Controller/1(err)
  Constant/1 -> PID_Controller/2(reset)
  PID_Controller/1(u) -> Saturation/1
  Saturation/1 -> Gain/1
  Gain/1 -> thetaD/1

== system our_ch47/Subsystem/直升机4 PID control/位置控制器/垂向速度控制器 ==
  VzD : Inport
  Vz : Inport  Port=2
  Constant : Constant  Value=0  OutDataTypeStr=Inherit: Inherit via back propagation
  Data Type Conversion : DataTypeConversion  OutDataTypeStr=double
  Gain : Gain  Gain=-1
  PID_Controller : Subsystem
  Saturation : Saturate  UpperLimit=8  LowerLimit=-6
  Subtract : Sum  Inputs=+-
  Sum : Sum  Inputs=|++
  hover_throttle : Constant  Value=x0(1)  OutDataTypeStr=Inherit: Inherit via back propagation
  Col : Outport  VectorParamsAs1DForOutWhenUnconnected=off
  wires:
  VzD/1 -> Subtract/1
  Vz/1 -> Subtract/2
  Subtract/1 -> PID_Controller/1(err)
  Constant/1 -> PID_Controller/2(reset)
  Data Type Conversion/1 -> Col/1
  hover_throttle/1 -> Sum/2
  PID_Controller/1(u) -> Saturation/1
  Saturation/1 -> Gain/1
  Sum/1 -> Data Type Conversion/1
  Gain/1 -> Sum/1

== system our_ch47/Subsystem/直升机4 PID control/位置控制器/高度控制器 ==
  设定高度 : Inport
  实际高度 : Inport  Port=2
  Data Type Conversion1 : DataTypeConversion  OutDataTypeStr=single  LockScale=on
  Data Type Conversion2 : DataTypeConversion  OutDataTypeStr=single  LockScale=on
  Data Type Conversion3 : DataTypeConversion  OutDataTypeStr=double  LockScale=on
  高度控制器H-A : Subsystem
  VzD : Outport
  wires:
  实际高度/1 -> Data Type Conversion2/1
  设定高度/1 -> Data Type Conversion1/1
  高度控制器H-A/1(VzD) -> Data Type Conversion3/1
  Data Type Conversion1/1 -> 高度控制器H-A/1(altitude_sp_m)
  Data Type Conversion2/1 -> 高度控制器H-A/2(altitude_m)
  Data Type Conversion3/1 -> VzD/1

== system our_ch47/Subsystem/直升机4 PID control/姿态控制器/俯仰控制器H-A ==
  PitchD : Inport
  Pitch : Inport  Port=2
  PitchRate : Inport  Port=3
  AltitudeV_Controller : Subsystem
  Data Type Conversion : DataTypeConversion  OutDataTypeStr=single  LockScale=on
  Data Type Conversion1 : DataTypeConversion  OutDataTypeStr=single  LockScale=on
  角度换 : Subsystem
  Lon : Outport  VectorParamsAs1DForOutWhenUnconnected=off
  wires:
  AltitudeV_Controller/1(Lon) -> Lon/1
  PitchRate/1 -> Data Type Conversion1/1
  Pitch/1 -> Data Type Conversion/1
  PitchD/1 -> 角度换/1(PitchD)
  Data Type Conversion/1 -> 角度换/2(Pitch)
  Data Type Conversion1/1 -> AltitudeV_Controller/2(PitchRate)
  角度换/1(PitchRateD) -> AltitudeV_Controller/1(PitchRateD)

== system our_ch47/Subsystem/直升机4 PID control/姿态控制器/滚转控制器H-A ==
  RollD : Inport
  Roll : Inport  Port=2
  RollRate : Inport  Port=3
  AltitudeV_Controller : Subsystem
  Altitude_Controller : Subsystem
  Data Type Conversion : DataTypeConversion  OutDataTypeStr=single  LockScale=on
  Data Type Conversion1 : DataTypeConversion  OutDataTypeStr=single  LockScale=on
  Lat : Outport  VectorParamsAs1DForOutWhenUnconnected=off
  wires:
  AltitudeV_Controller/1(Lat) -> Lat/1  "lat"
  RollRate/1 -> Data Type Conversion1/1
  Roll/1 -> Data Type Conversion/1
  Data Type Conversion/1 -> Altitude_Controller/2(Roll)
  Data Type Conversion1/1 -> AltitudeV_Controller/2(RollRate)
  RollD/1 -> Altitude_Controller/1(RollD)
  Altitude_Controller/1(RollRateD) -> AltitudeV_Controller/1(RollRateD)

== system our_ch47/Subsystem/直升机4 PID control/姿态控制器/航向控制器H-A ==
  YawD : Inport
  Yaw : Inport  Port=2
  YawRate : Inport  Port=3
  AltitudeV_Controller : Subsystem
  Altitude_Controller : Subsystem
  Data Type Conversion : DataTypeConversion  OutDataTypeStr=single  LockScale=on
  Data Type Conversion1 : DataTypeConversion  OutDataTypeStr=single  LockScale=on
  Ped : Outport  VectorParamsAs1DForOutWhenUnconnected=off
  wires:
  AltitudeV_Controller/1(Ped) -> Ped/1
  YawRate/1 -> Data Type Conversion1/1
  Yaw/1 -> Data Type Conversion/1
  YawD/1 -> Altitude_Controller/1(YawD)
  Data Type Conversion/1 -> Altitude_Controller/2(Yaw)
  Data Type Conversion1/1 -> AltitudeV_Controller/2(YawRate)
  Altitude_Controller/1(YawRateD) -> AltitudeV_Controller/1(YawRateD)

== system our_ch47/Subsystem/直升机1 PID control/位置控制器/侧向位置控制器/侧向位置控制器 ==
  yd_m : Inport
  y_m : Inport  Port=2
  Constant : Constant  Value=0  OutDataTypeStr=Inherit: Inherit via back propagation
  PID_Controller : Subsystem
  Saturation : Saturate  UpperLimit=10  LowerLimit=-10
  Saturation1 : Saturate  UpperLimit=10  LowerLimit=-10
  Subtract : Sum  Inputs=+-
  VyD : Outport  VectorParamsAs1DForOutWhenUnconnected=off
  wires:
  Saturation1/1 -> PID_Controller/1(err)
  Subtract/1 -> Saturation1/1
  PID_Controller/1(u) -> Saturation/1
  Saturation/1 -> VyD/1
  Constant/1 -> PID_Controller/2(reset)
  y_m/1 -> Subtract/2
  yd_m/1 -> Subtract/1

== system our_ch47/Subsystem/直升机1 PID control/位置控制器/侧向速度控制器/PID_Controller ==
  err : Inport
  reset : Inport  Port=2
  Add : Sum
  I_Control : Subsystem  mask{ki=PID_Param1.Ki_Vy, max_i=0.3, min_i=-0.3}
  P_Control : Subsystem  mask{kp=PID_Param1.Kp_Vy}
  u : Outport  VectorParamsAs1DForOutWhenUnconnected=off
  wires:
  Add/1 -> u/1
  I_Control/1(i_out) -> Add/2
  P_Control/1(p_out) -> Add/1
  reset/1 -> I_Control/2(reset)
  err/1 -> I_Control/1(err), P_Control/1(err)

== system our_ch47/Subsystem/直升机1 PID control/位置控制器/前向位置控制器/前向位置控制器 ==
  xd_m : Inport
  x_m : Inport  Port=2
  Constant : Constant  Value=0  OutDataTypeStr=Inherit: Inherit via back propagation
  PID_Controller : Subsystem
  Saturation : Saturate  UpperLimit=12  LowerLimit=-12
  Saturation1 : Saturate  UpperLimit=10  LowerLimit=-10
  Subtract : Sum  Inputs=+-
  VxD : Outport  VectorParamsAs1DForOutWhenUnconnected=off
  wires:
  xd_m/1 -> Subtract/1
  x_m/1 -> Subtract/2
  Constant/1 -> PID_Controller/2(reset)
  Saturation/1 -> VxD/1
  PID_Controller/1(u) -> Saturation/1
  Subtract/1 -> Saturation1/1
  Saturation1/1 -> PID_Controller/1(err)

== system our_ch47/Subsystem/直升机1 PID control/位置控制器/前向速度控制器/PID_Controller ==
  err : Inport
  reset : Inport  Port=2
  Add : Sum
  I_Control : Subsystem  mask{ki=PID_Param1.Ki_Vx, max_i=0.3, min_i=-0.3}
  P_Control : Subsystem  mask{kp=PID_Param1.Kp_Vx}
  u : Outport  VectorParamsAs1DForOutWhenUnconnected=off
  wires:
  err/1 -> P_Control/1(err), I_Control/1(err)
  reset/1 -> I_Control/2(reset)
  P_Control/1(p_out) -> Add/1
  I_Control/1(i_out) -> Add/2
  Add/1 -> u/1

== system our_ch47/Subsystem/直升机1 PID control/位置控制器/垂向速度控制器/PID_Controller ==
  err : Inport
  reset : Inport  Port=2
  Add : Sum
  I_Control : Subsystem  mask{ki=PID_Param1.Ki_Vz, max_i=0.3, min_i=-0.3}
  P_Control : Subsystem  mask{kp=PID_Param1.Kp_Vz}
  u : Outport  VectorParamsAs1DForOutWhenUnconnected=off
  wires:
  err/1 -> P_Control/1(err), I_Control/1(err)
  reset/1 -> I_Control/2(reset)
  P_Control/1(p_out) -> Add/1
  I_Control/1(i_out) -> Add/2
  Add/1 -> u/1

== system our_ch47/Subsystem/直升机1 PID control/位置控制器/高度控制器/高度控制器H-A ==
  altitude_sp_m : Inport
  altitude_m : Inport  Port=2
  Constant : Constant  Value=0  OutDataTypeStr=Inherit: Inherit via back propagation
  PID_Controller : Subsystem
  Saturation : Saturate  UpperLimit=2  LowerLimit=-2
  Saturation1 : Saturate  UpperLimit=10  LowerLimit=-10
  Subtract : Sum  Inputs=+-
  VzD : Outport  VectorParamsAs1DForOutWhenUnconnected=off
  wires:
  altitude_sp_m/1 -> Subtract/1
  altitude_m/1 -> Subtract/2
  Constant/1 -> PID_Controller/2(reset)
  Saturation/1 -> VzD/1
  PID_Controller/1(u) -> Saturation/1
  Subtract/1 -> Saturation1/1
  Saturation1/1 -> PID_Controller/1(err)

== system our_ch47/Subsystem/直升机1 PID control/姿态控制器/俯仰控制器H-A/AltitudeV_Controller ==
  PitchRateD : Inport
  PitchRate : Inport  Port=2
  PID_Controller : Subsystem
  Saturation : Saturate  UpperLimit=5  LowerLimit=-5
  Subtract : Sum  Inputs=+-
  Lon : Outport  VectorParamsAs1DForOutWhenUnconnected=off
  wires:
  PitchRateD/1 -> Subtract/1
  PitchRate/1 -> Subtract/2
  Subtract/1 -> PID_Controller/1(err)
  Saturation/1 -> Lon/1
  PID_Controller/1(u) -> Saturation/1

== system our_ch47/Subsystem/直升机1 PID control/姿态控制器/俯仰控制器H-A/角度换 ==
  PitchD : Inport
  Pitch : Inport  Port=2
  PID_Controller : Subsystem
  Saturation : Saturate  UpperLimit=45  LowerLimit=-45
  Saturation1 : Saturate  UpperLimit=45  LowerLimit=-45
  Subtract : Sum  Inputs=+-
  PitchRateD : Outport  VectorParamsAs1DForOutWhenUnconnected=off
  wires:
  PitchD/1 -> Subtract/1
  Pitch/1 -> Subtract/2
  PID_Controller/1(u) -> Saturation/1
  Saturation1/1 -> PID_Controller/1(err)
  Subtract/1 -> Saturation1/1
  Saturation/1 -> PitchRateD/1

== system our_ch47/Subsystem/直升机1 PID control/姿态控制器/滚转控制器H-A/AltitudeV_Controller ==
  RollRateD : Inport
  RollRate : Inport  Port=2
  Constant : Constant  Value=0  OutDataTypeStr=Inherit: Inherit via back propagation
  PID_Controller : Subsystem
  Saturation : Saturate  UpperLimit=5  LowerLimit=-5
  Subtract : Sum  Inputs=+-
  Lat : Outport  VectorParamsAs1DForOutWhenUnconnected=off
  wires:
  RollRateD/1 -> Subtract/1
  RollRate/1 -> Subtract/2
  Subtract/1 -> PID_Controller/1(err)
  Constant/1 -> PID_Controller/2(reset)
  Saturation/1 -> Lat/1
  PID_Controller/1(u) -> Saturation/1

== system our_ch47/Subsystem/直升机1 PID control/姿态控制器/滚转控制器H-A/Altitude_Controller ==
  RollD : Inport
  Roll : Inport  Port=2
  PID_Controller : Subsystem
  Saturation : Saturate  UpperLimit=45  LowerLimit=-45
  Saturation1 : Saturate  UpperLimit=45  LowerLimit=-45
  Subtract : Sum  Inputs=+-
  RollRateD : Outport  VectorParamsAs1DForOutWhenUnconnected=off
  wires:
  RollD/1 -> Subtract/1
  Roll/1 -> Subtract/2
  Saturation/1 -> RollRateD/1
  PID_Controller/1(u) -> Saturation/1
  Subtract/1 -> Saturation1/1
  Saturation1/1 -> PID_Controller/1(err)

== system our_ch47/Subsystem/直升机1 PID control/姿态控制器/航向控制器H-A/AltitudeV_Controller ==
  YawRateD : Inport
  YawRate : Inport  Port=2
  Constant : Constant  Value=0  OutDataTypeStr=Inherit: Inherit via back propagation
  Controller : Subsystem
  Saturation : Saturate  UpperLimit=5  LowerLimit=-5
  Subtract : Sum  Inputs=+-
  Ped : Outport  VectorParamsAs1DForOutWhenUnconnected=off
  wires:
  YawRateD/1 -> Subtract/1
  YawRate/1 -> Subtract/2
  Subtract/1 -> Controller/1(err)
  Constant/1 -> Controller/2(reset)
  Saturation/1 -> Ped/1
  Controller/1(u) -> Saturation/1

== system our_ch47/Subsystem/直升机1 PID control/姿态控制器/航向控制器H-A/Altitude_Controller ==
  YawD : Inport
  Yaw : Inport  Port=2
  Constant : Constant  Value=0  OutDataTypeStr=Inherit: Inherit via back propagation
  Controller : Subsystem
  Saturation : Saturate  UpperLimit=45  LowerLimit=-45
  Saturation1 : Saturate  UpperLimit=45  LowerLimit=-45
  Subtract : Sum  Inputs=+-
  YawRateD : Outport  VectorParamsAs1DForOutWhenUnconnected=off
  wires:
  YawD/1 -> Subtract/1
  Yaw/1 -> Subtract/2
  Constant/1 -> Controller/2(reset)
  Saturation/1 -> YawRateD/1
  Controller/1(u) -> Saturation/1
  Subtract/1 -> Saturation1/1
  Saturation1/1 -> Controller/1(err)

== system our_ch47/Subsystem/直升机2 PID control/位置控制器/侧向位置控制器/侧向位置控制器 ==
  yd_m : Inport
  y_m : Inport  Port=2
  Constant : Constant  Value=0  OutDataTypeStr=Inherit: Inherit via back propagation
  PID_Controller : Subsystem
  Saturation : Saturate  UpperLimit=10  LowerLimit=-10
  Saturation1 : Saturate  UpperLimit=10  LowerLimit=-10
  Subtract : Sum  Inputs=+-
  VyD : Outport  VectorParamsAs1DForOutWhenUnconnected=off
  wires:
  Saturation1/1 -> PID_Controller/1(err)
  Subtract/1 -> Saturation1/1
  PID_Controller/1(u) -> Saturation/1
  Saturation/1 -> VyD/1
  Constant/1 -> PID_Controller/2(reset)
  y_m/1 -> Subtract/2
  yd_m/1 -> Subtract/1

== system our_ch47/Subsystem/直升机2 PID control/位置控制器/侧向速度控制器/PID_Controller ==
  err : Inport
  reset : Inport  Port=2
  Add : Sum
  I_Control : Subsystem  mask{ki=PID_Param1.Ki_Vy, max_i=0.3, min_i=-0.3}
  P_Control : Subsystem  mask{kp=PID_Param1.Kp_Vy}
  u : Outport  VectorParamsAs1DForOutWhenUnconnected=off
  wires:
  Add/1 -> u/1
  I_Control/1(i_out) -> Add/2
  P_Control/1(p_out) -> Add/1
  reset/1 -> I_Control/2(reset)
  err/1 -> I_Control/1(err), P_Control/1(err)

== system our_ch47/Subsystem/直升机2 PID control/位置控制器/前向位置控制器/前向位置控制器 ==
  xd_m : Inport
  x_m : Inport  Port=2
  Constant : Constant  Value=0  OutDataTypeStr=Inherit: Inherit via back propagation
  PID_Controller : Subsystem
  Saturation : Saturate  UpperLimit=12  LowerLimit=-12
  Saturation1 : Saturate  UpperLimit=10  LowerLimit=-10
  Subtract : Sum  Inputs=+-
  VxD : Outport  VectorParamsAs1DForOutWhenUnconnected=off
  wires:
  xd_m/1 -> Subtract/1
  x_m/1 -> Subtract/2
  Constant/1 -> PID_Controller/2(reset)
  Saturation/1 -> VxD/1
  PID_Controller/1(u) -> Saturation/1
  Subtract/1 -> Saturation1/1
  Saturation1/1 -> PID_Controller/1(err)

== system our_ch47/Subsystem/直升机2 PID control/位置控制器/前向速度控制器/PID_Controller ==
  err : Inport
  reset : Inport  Port=2
  Add : Sum
  I_Control : Subsystem  mask{ki=PID_Param1.Ki_Vx, max_i=0.3, min_i=-0.3}
  P_Control : Subsystem  mask{kp=PID_Param1.Kp_Vx}
  u : Outport  VectorParamsAs1DForOutWhenUnconnected=off
  wires:
  err/1 -> P_Control/1(err), I_Control/1(err)
  reset/1 -> I_Control/2(reset)
  P_Control/1(p_out) -> Add/1
  I_Control/1(i_out) -> Add/2
  Add/1 -> u/1

== system our_ch47/Subsystem/直升机2 PID control/位置控制器/垂向速度控制器/PID_Controller ==
  err : Inport
  reset : Inport  Port=2
  Add : Sum
  I_Control : Subsystem  mask{ki=PID_Param1.Ki_Vz, max_i=0.3, min_i=-0.3}
  P_Control : Subsystem  mask{kp=PID_Param1.Kp_Vz}
  u : Outport  VectorParamsAs1DForOutWhenUnconnected=off
  wires:
  err/1 -> P_Control/1(err), I_Control/1(err)
  reset/1 -> I_Control/2(reset)
  P_Control/1(p_out) -> Add/1
  I_Control/1(i_out) -> Add/2
  Add/1 -> u/1

== system our_ch47/Subsystem/直升机2 PID control/位置控制器/高度控制器/高度控制器H-A ==
  altitude_sp_m : Inport
  altitude_m : Inport  Port=2
  Constant : Constant  Value=0  OutDataTypeStr=Inherit: Inherit via back propagation
  PID_Controller : Subsystem
  Saturation : Saturate  UpperLimit=2  LowerLimit=-2
  Saturation1 : Saturate  UpperLimit=10  LowerLimit=-10
  Subtract : Sum  Inputs=+-
  VzD : Outport  VectorParamsAs1DForOutWhenUnconnected=off
  wires:
  altitude_sp_m/1 -> Subtract/1
  altitude_m/1 -> Subtract/2
  Constant/1 -> PID_Controller/2(reset)
  Saturation/1 -> VzD/1
  PID_Controller/1(u) -> Saturation/1
  Subtract/1 -> Saturation1/1
  Saturation1/1 -> PID_Controller/1(err)

== system our_ch47/Subsystem/直升机2 PID control/姿态控制器/俯仰控制器H-A/AltitudeV_Controller ==
  PitchRateD : Inport
  PitchRate : Inport  Port=2
  PID_Controller : Subsystem
  Saturation : Saturate  UpperLimit=5  LowerLimit=-5
  Subtract : Sum  Inputs=+-
  Lon : Outport  VectorParamsAs1DForOutWhenUnconnected=off
  wires:
  PitchRateD/1 -> Subtract/1
  PitchRate/1 -> Subtract/2
  Subtract/1 -> PID_Controller/1(err)
  Saturation/1 -> Lon/1
  PID_Controller/1(u) -> Saturation/1

== system our_ch47/Subsystem/直升机2 PID control/姿态控制器/俯仰控制器H-A/角度换 ==
  PitchD : Inport
  Pitch : Inport  Port=2
  PID_Controller : Subsystem
  Saturation : Saturate  UpperLimit=45  LowerLimit=-45
  Saturation1 : Saturate  UpperLimit=45  LowerLimit=-45
  Subtract : Sum  Inputs=+-
  PitchRateD : Outport  VectorParamsAs1DForOutWhenUnconnected=off
  wires:
  PitchD/1 -> Subtract/1
  Pitch/1 -> Subtract/2
  PID_Controller/1(u) -> Saturation/1
  Saturation1/1 -> PID_Controller/1(err)
  Subtract/1 -> Saturation1/1
  Saturation/1 -> PitchRateD/1

== system our_ch47/Subsystem/直升机2 PID control/姿态控制器/滚转控制器H-A/AltitudeV_Controller ==
  RollRateD : Inport
  RollRate : Inport  Port=2
  Constant : Constant  Value=0  OutDataTypeStr=Inherit: Inherit via back propagation
  PID_Controller : Subsystem
  Saturation : Saturate  UpperLimit=5  LowerLimit=-5
  Subtract : Sum  Inputs=+-
  Lat : Outport  VectorParamsAs1DForOutWhenUnconnected=off
  wires:
  RollRateD/1 -> Subtract/1
  RollRate/1 -> Subtract/2
  Subtract/1 -> PID_Controller/1(err)
  Constant/1 -> PID_Controller/2(reset)
  Saturation/1 -> Lat/1
  PID_Controller/1(u) -> Saturation/1

== system our_ch47/Subsystem/直升机2 PID control/姿态控制器/滚转控制器H-A/Altitude_Controller ==
  RollD : Inport
  Roll : Inport  Port=2
  PID_Controller : Subsystem
  Saturation : Saturate  UpperLimit=45  LowerLimit=-45
  Saturation1 : Saturate  UpperLimit=45  LowerLimit=-45
  Subtract : Sum  Inputs=+-
  RollRateD : Outport  VectorParamsAs1DForOutWhenUnconnected=off
  wires:
  RollD/1 -> Subtract/1
  Roll/1 -> Subtract/2
  Saturation/1 -> RollRateD/1
  PID_Controller/1(u) -> Saturation/1
  Subtract/1 -> Saturation1/1
  Saturation1/1 -> PID_Controller/1(err)

== system our_ch47/Subsystem/直升机2 PID control/姿态控制器/航向控制器H-A/AltitudeV_Controller ==
  YawRateD : Inport
  YawRate : Inport  Port=2
  Constant : Constant  Value=0  OutDataTypeStr=Inherit: Inherit via back propagation
  Controller : Subsystem
  Saturation : Saturate  UpperLimit=5  LowerLimit=-5
  Subtract : Sum  Inputs=+-
  Ped : Outport  VectorParamsAs1DForOutWhenUnconnected=off
  wires:
  YawRateD/1 -> Subtract/1
  YawRate/1 -> Subtract/2
  Subtract/1 -> Controller/1(err)
  Constant/1 -> Controller/2(reset)
  Saturation/1 -> Ped/1
  Controller/1(u) -> Saturation/1
